simulink model "powerwindow_tl_v01"  (R2021a)
settings: Solver=ode1  StartTime=0.0  StopTime=20.0  FixedStep=0.01  RelTol=1e-3
PreLoadFcn:
  | if exist('tl_preloadfcn','file'), tl_preloadfcn(gcs,'22.1.0.27'); end
PostLoadFcn:
  | if exist('tl_postloadfcn','file'), tl_postloadfcn(gcs,'22.1.0.27'); end
InitFcn:
  | if exist('tlds_init','file'), tlds_init(gcs); end
StartFcn:
  | if exist('tlds_start','file'), tlds_start(gcs); end
StopFcn:
  | if exist('tlds_stop','file'), tlds_stop(gcs); end
undefined symbols (not defined in the file): auto_down_time, auto_up_time, emergency_down_time, position_endstop_top
libraries: tllib x7
(part 1 of 2)
PreSaveFcn:
  | if exist('tl_presavefcn','file'), tl_presavefcn(gcs); end
CloseFcn:
  | if exist('tl_closefcn','file'), tl_closefcn(gcs); end
settings Model: TL_MAIN_DATA={'codeopt',{'cleancode',1},'date',738946.6177900926,'advcodeopt',{'ExtendedBlockComments';'true'}}  DS_PROJECTFILE=powerwindow_tl_v01.dd  TLVersion=22.1.0.27  TL_GLOBAL_LOGGING_MODE=4  Creator=Wolfgang Meincke  LastModifiedBy=yatishc
settings SolverCC: AlgebraicLoopSolver=TrustRegion
settings DataIOCC: LimitDataPoints=on  SaveFormat=Array  ReturnWorkspaceOutputs=off
settings OptimizationCC: BlockReduction=off  BooleanDataType=off  ConditionallyExecuteInputs=off  OptimizeBlockIOStorage=off  BufferReuse=off  GlobalBufferReuse=off  ExpressionFolding=off  ExpressionDepthLimit=2147483647  LocalBlockOutputs=off  LifeSpan=inf  OptimizeDataStoreBuffers=off  BusAssignmentInplaceUpdate=off
settings DebuggingCC: SaveWithParameterizedLinksMsg=none  UnderspecifiedInitializationDetection=Classic  MergeDetectMultiDrivingBlocksExec=none  MultiTaskDSMMsg=warning  MultiTaskCondExecSysMsg=none  FcnCallInpInsideContextMsg=warning  UnconnectedInputMsg=none  UnconnectedOutputMsg=none  BusObjectLabelMismatch=error  StateNameClashWarn=warning  StrictBusMsg=ErrorOnBusTreatedAsVector  NonBusSignalsTreatedAsBus=error  SFUnexpectedBacktrackingDiag=warning  SFNoUnconditionalDefaultTransitionDiag=warning  SFMachineParentedDataDiag=warning  ArithmeticOperatorsInVariantConditions=warning
settings HardwareCC: ProdBitPerPointer=32  ProdBitPerSizeT=32  ProdBitPerPtrDiffT=32  ProdLargestAtomicFloat=None  ProdIntDivRoundTo=Undefined  ProdEndianess=Unspecified  ProdWordSize=32  ProdHWDeviceType=32-bit Generic
settings ModelReferenceCC: PropagateSignalLabelsOutOfModel=off
settings SFSimCC: SimUseLocalCustomCode=off  SimParseCustomCode=off  CustomCodeUndefinedFunction=UseInterfaceOnly
settings RTWCC: RTWUseLocalCustomCode=off
settings CodeAppCC: StateflowObjectComments=on
settings GRTTargetCC: TargetLangStandard=C89/C90 (ANSI)  CombineOutputUpdateFcns=off  GRTInterface=on
settings ConfigComp: CovMetricSettings=dw  CovSaveCumulativeToWorkspaceVar=on  CovSaveSingleToWorkspaceVar=on  CovExternalEMLEnable=off  CovSFcnEnable=off

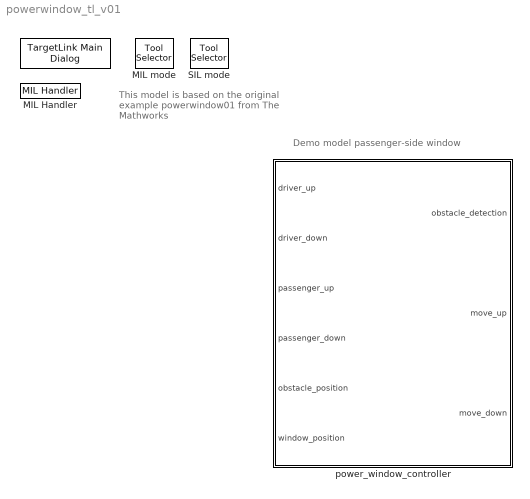
== system powerwindow_tl_v01 ==
  note: Demo model passenger-side window
  note: This model is based on the
      | original example powerwindow01
      | from The Mathworks
  " " : tllib/TargetLink Main Dialog  data=[]
      settings: SourceProductName=dSPACE TargetLink common blockset
  MIL Handler : tllib/MIL Handler  data={'date',730486}
      settings: SourceProductName=dSPACE TargetLink common blockset
  MIL mode : tllib/Tool Selector  Description=MIL\nmode  data={'date',730486}
      settings: SourceProductName=dSPACE TargetLink common blockset
  SIL mode : tllib/Tool Selector  Description=SIL\nmode  data={'date',730486}
      settings: SourceProductName=dSPACE TargetLink common blockset
  power_window_controller : Subsystem  Tag=TargetLink Simulation Frame  mask(TL_SimFrame){}
      settings: CopyFcn=if exist('tl_copyfcn','file'), tl_copyfcn(gcbh); end  NameChangeFcn=if exist('tl_framenamechangefcn','file'), tl_framenamechangefcn(gcbh); end
      settings: OpenFcn=|
      | if exist('open_tlsubsystem','file')
      |    open_tlsubsystem(gcbh);
      | else
      |    tlsubsystem = ...
      |       find_system(gcb, ...
      |       'LookUnderMasks','on', ...
      |       'FollowLinks','on', ...
      |       'Tag','MIL Subsystem');
      |    open_system(tlsubsystem);
      | end
      mask Display: disp('TargetLink\nModel-\nin-the-loop\nmode')

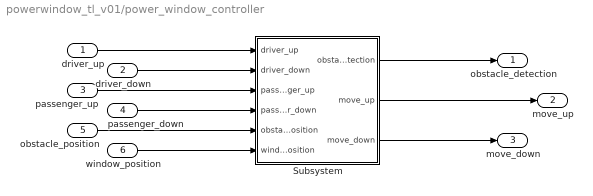
== system powerwindow_tl_v01/power_window_controller ==
  driver_up : Inport
  driver_down : Inport  Port=2
  passenger_up : Inport  Port=3
  passenger_down : Inport  Port=4
  obstacle_position : Inport  Port=5
  window_position : Inport  Port=6
  Subsystem : Subsystem  Tag=struct('sfcnName','power_window_controller_sf','subFunction','','srcSubsystem','')  mask(TL_Enable){}
      settings: OpenFcn=warndlg(get_param(gcb,'MaskHelp'),'Serious Warning');
      mask Help: This subsystem keeps the TargetLink subsystem (subsystem with TargetLink blocks for production code generation), and is needed for the TargetLink simulation frame to work properly. DO NOT DELETE OR MODIFY IT!
  obstacle_detection : Outport  VectorParamsAs1DForOutWhenUnconnected=off
  move_up : Outport  Port=2  VectorParamsAs1DForOutWhenUnconnected=off
  move_down : Outport  Port=3  VectorParamsAs1DForOutWhenUnconnected=off
  wires:
  driver_up/1 -> Subsystem/1(driver_up)
  driver_down/1 -> Subsystem/2(driver_down)
  passenger_up/1 -> Subsystem/3(passenger_up)
  passenger_down/1 -> Subsystem/4(passenger_down)
  obstacle_position/1 -> Subsystem/5(obstacle_position)
  window_position/1 -> Subsystem/6(window_position)
  Subsystem/1(obstacle_detection) -> obstacle_detection/1
  Subsystem/2(move_up) -> move_up/1
  Subsystem/3(move_down) -> move_down/1

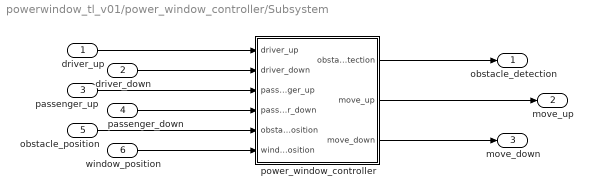
== system powerwindow_tl_v01/power_window_controller/Subsystem ==
  driver_up : Inport
  driver_down : Inport  Port=2
  passenger_up : Inport  Port=3
  passenger_down : Inport  Port=4
  obstacle_position : Inport  Port=5
  window_position : Inport  Port=6
  power_window_controller : Subsystem  Tag=MIL Subsystem  Description=a  RequirementInfo={} %GIDa_b80cfd7f_fc3d_42d1_9879_5951100bdf27  LoadFcn=|
      | if exist('TargetLink.SimFrameHandler.TLSubsystem','class')
      |     TargetLink.SimFrameHandler.TLSubsystem.CreateWatchDog(gcbh);
      | end
      settings: CopyFcn=if exist('tl_copyfcn','file'), tl_copyfcn(gcbh); end  NameChangeFcn=if exist('tl_namechangefcn','file'), tl_namechangefcn(gcbh); end  DestroyFcn=if exist('update_tl_main_dlg','file'), update_tl_main_dlg('TL_subs_display'); end
      mask Display: disp('TargetLink Subsystem')
  obstacle_detection : Outport  VectorParamsAs1DForOutWhenUnconnected=off
  move_up : Outport  Port=2  VectorParamsAs1DForOutWhenUnconnected=off
  move_down : Outport  Port=3  VectorParamsAs1DForOutWhenUnconnected=off
  wires:
  driver_up/1 -> power_window_controller/1(driver_up)
  driver_down/1 -> power_window_controller/2(driver_down)
  passenger_up/1 -> power_window_controller/3(passenger_up)
  passenger_down/1 -> power_window_controller/4(passenger_down)
  obstacle_position/1 -> power_window_controller/5(obstacle_position)
  window_position/1 -> power_window_controller/6(window_position)
  power_window_controller/1(obstacle_detection) -> obstacle_detection/1
  power_window_controller/2(move_up) -> move_up/1
  power_window_controller/3(move_down) -> move_down/1

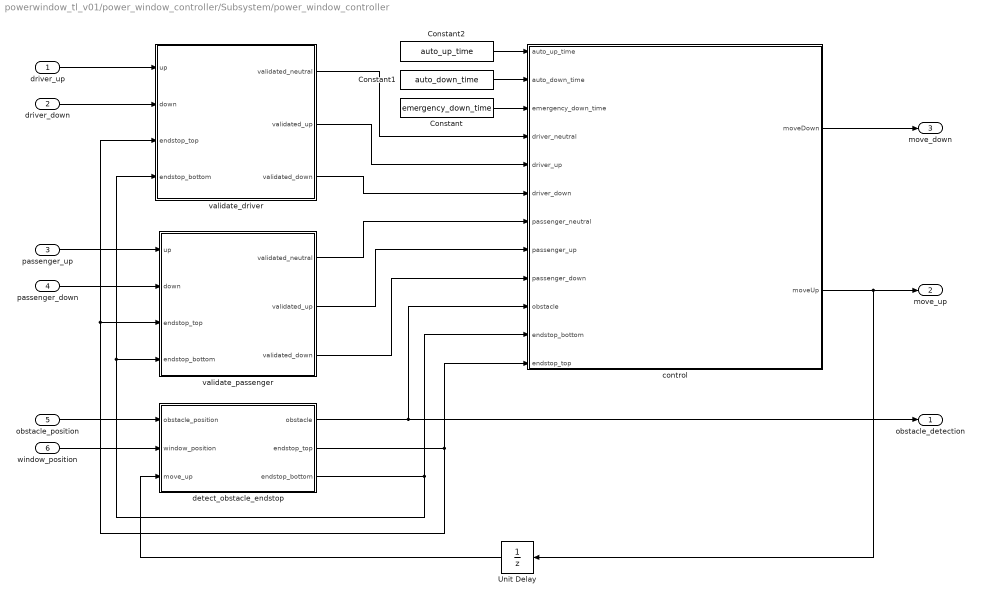
== system powerwindow_tl_v01/power_window_controller/Subsystem/power_window_controller ==
  driver_up : Inport  RequirementInfo={} %GIDa_750a3b1c_a79a_4067_88d9_431790a89f5d  PortDimensions=1  mask(TL_Inport){data={'output',{'variable','Interface_Variables/driver_up'},'date',737859.74382688652}}
      settings: CopyFcn=if exist('copy_tlblock','file')==2,copy_tlblock(gcbh);end  DeleteFcn=if exist('delete_tlblock','file')==2,delete_tlblock(gcbh);end  NameChangeFcn=if exist('rename_tlblock','file')==2,rename_tlblock(gcbh);end  OpenFcn=if exist('tl_open_blockdlg','file')==2,tl_open_blockdlg(gcbh);else,open_system(gcbh,'parameter');end
      mask Help: eval(['if exist(''tl_online_help'',''file'') == 2, tl_online_help(''Topic'',''TL_Inport''),else, web([''jar:file:///'',matlabroot,''/help/toolbox/simulink/help.jar!/slref/' lower(get_param(gcbh,'Blocktype')) '.html''], ''-helpbrowser''),end'])
      mask Display:
      | [x,y] = tlDrawBrandOnBlockIcon(gcbh);
      | plot(x,y);
  driver_down : Inport  RequirementInfo={} %GIDa_6d11f596_882a_4ff9_a83e_d4d289160ffc  Port=2  PortDimensions=1  mask(TL_Inport){data={'output',{'variable','Interface_Variables/driver_down'},'date',737859.74382813659}}
      settings: CopyFcn=if exist('copy_tlblock','file')==2,copy_tlblock(gcbh);end  DeleteFcn=if exist('delete_tlblock','file')==2,delete_tlblock(gcbh);end  NameChangeFcn=if exist('rename_tlblock','file')==2,rename_tlblock(gcbh);end  OpenFcn=if exist('tl_open_blockdlg','file')==2,tl_open_blockdlg(gcbh);else,open_system(gcbh,'parameter');end
      mask Help: eval(['if exist(''tl_online_help'',''file'') == 2, tl_online_help(''Topic'',''TL_Inport''),else, web([''jar:file:///'',matlabroot,''/help/toolbox/simulink/help.jar!/slref/' lower(get_param(gcbh,'Blocktype')) '.html''], ''-helpbrowser''),end'])
      mask Display:
      | [x,y] = tlDrawBrandOnBlockIcon(gcbh);
      | plot(x,y);
  passenger_up : Inport  RequirementInfo={} %GIDa_37c1ad15_e81b_4888_89b1_052434cfbb89  Port=3  PortDimensions=1  mask(TL_Inport){data={'output',{'variable','Interface_Variables/passenger_up'},'date',737859.74382853007}}
      settings: CopyFcn=if exist('copy_tlblock','file')==2,copy_tlblock(gcbh);end  DeleteFcn=if exist('delete_tlblock','file')==2,delete_tlblock(gcbh);end  NameChangeFcn=if exist('rename_tlblock','file')==2,rename_tlblock(gcbh);end  OpenFcn=if exist('tl_open_blockdlg','file')==2,tl_open_blockdlg(gcbh);else,open_system(gcbh,'parameter');end
      mask Help: eval(['if exist(''tl_online_help'',''file'') == 2, tl_online_help(''Topic'',''TL_Inport''),else, web([''jar:file:///'',matlabroot,''/help/toolbox/simulink/help.jar!/slref/' lower(get_param(gcbh,'Blocktype')) '.html''], ''-helpbrowser''),end'])
      mask Display:
      | [x,y] = tlDrawBrandOnBlockIcon(gcbh);
      | plot(x,y);
  passenger_down : Inport  RequirementInfo={} %GIDa_785e7f27_a7f1_4b54_8fd7_681828111c23  Port=4  PortDimensions=1  mask(TL_Inport){data={'output',{'variable','Interface_Variables/passenger_down'},'date',737859.74382914347}}
      settings: CopyFcn=if exist('copy_tlblock','file')==2,copy_tlblock(gcbh);end  DeleteFcn=if exist('delete_tlblock','file')==2,delete_tlblock(gcbh);end  NameChangeFcn=if exist('rename_tlblock','file')==2,rename_tlblock(gcbh);end  OpenFcn=if exist('tl_open_blockdlg','file')==2,tl_open_blockdlg(gcbh);else,open_system(gcbh,'parameter');end
      mask Help: eval(['if exist(''tl_online_help'',''file'') == 2, tl_online_help(''Topic'',''TL_Inport''),else, web([''jar:file:///'',matlabroot,''/help/toolbox/simulink/help.jar!/slref/' lower(get_param(gcbh,'Blocktype')) '.html''], ''-helpbrowser''),end'])
      mask Display:
      | [x,y] = tlDrawBrandOnBlockIcon(gcbh);
      | plot(x,y);
  obstacle_position : Inport  RequirementInfo={} %GIDa_c852d148_69a2_44b2_91eb_10d8d3731c30  Port=5  PortDimensions=1  mask(TL_Inport){data={'output',{'variable','Interface_Variables/obstacle_position'},'autoscaling',{'mode',0},'date',737869.45975795144}}
      settings: CopyFcn=if exist('copy_tlblock','file')==2,copy_tlblock(gcbh);end  DeleteFcn=if exist('delete_tlblock','file')==2,delete_tlblock(gcbh);end  NameChangeFcn=if exist('rename_tlblock','file')==2,rename_tlblock(gcbh);end  OpenFcn=if exist('tl_open_blockdlg','file')==2,tl_open_blockdlg(gcbh);else,open_system(gcbh,'parameter');end
      mask Help: eval(['if exist(''tl_online_help'',''file'') == 2, tl_online_help(''Topic'',''TL_Inport''),else, web([''jar:file:///'',matlabroot,''/help/toolbox/simulink/help.jar!/slref/' lower(get_param(gcbh,'Blocktype')) '.html''], ''-helpbrowser''),end'])
      mask Display:
      | [x,y] = tlDrawBrandOnBlockIcon(gcbh);
      | plot(x,y);
  window_position : Inport  RequirementInfo={} %GIDa_527401dc_d2fc_43f1_9503_1f5713b1657a  Port=6  PortDimensions=1  mask(TL_Inport){data={'output',{'variable','Interface_Variables/window_position'},'autoscaling',{'mode',0},'date',738946.61777480319}}
      settings: CopyFcn=if exist('copy_tlblock','file')==2,copy_tlblock(gcbh);end  DeleteFcn=if exist('delete_tlblock','file')==2,delete_tlblock(gcbh);end  NameChangeFcn=if exist('rename_tlblock','file')==2,rename_tlblock(gcbh);end  OpenFcn=if exist('tl_open_blockdlg','file')==2,tl_open_blockdlg(gcbh);else,open_system(gcbh,'parameter');end
      mask Help: eval(['if exist(''tl_online_help'',''file'') == 2, tl_online_help(''Topic'',''TL_Inport''),else, web([''jar:file:///'',matlabroot,''/help/toolbox/simulink/help.jar!/slref/' lower(get_param(gcbh,'Blocktype')) '.html''], ''-helpbrowser''),end'])
      mask Display:
      | [x,y] = tlDrawBrandOnBlockIcon(gcbh);
      | plot(x,y);
  Constant : Constant  RequirementInfo={} %GIDa_c9ec6c8d_2743_4165_a701_f3b966281310  Value=emergency_down_time  mask(TL_Constant){data={'output',{'variable','Parameter/emergency_down_time'},'date',735993.41955673613}}
      settings: CopyFcn=if exist('copy_tlblock','file')==2,copy_tlblock(gcbh);end  DeleteFcn=if exist('delete_tlblock','file')==2,delete_tlblock(gcbh);end  NameChangeFcn=if exist('rename_tlblock','file')==2,rename_tlblock(gcbh);end  OpenFcn=if exist('tl_open_blockdlg','file')==2,tl_open_blockdlg(gcbh);else,open_system(gcbh,'parameter');end
      mask Help: eval(['if exist(''tl_online_help'',''file'') == 2, tl_online_help(''Topic'',''TL_Constant''),else, web([''jar:file:///'',matlabroot,''/help/toolbox/simulink/help.jar!/slref/' lower(get_param(gcbh,'Blocktype')) '.html''], ''-helpbrowser''),end'])
      mask Display:
      | [x,y] = tlDrawBrandOnBlockIcon(gcbh);
      | plot(x,y);
  Constant1 : Constant  RequirementInfo={} %GIDa_5bcfbdf2_6dc9_458c_8155_820a7ffe3dc3  Value=auto_down_time  mask(TL_Constant){data={'output',{'variable','Parameter/auto_down_time'},'date',735993.41940997681}}
      settings: CopyFcn=if exist('copy_tlblock','file')==2,copy_tlblock(gcbh);end  DeleteFcn=if exist('delete_tlblock','file')==2,delete_tlblock(gcbh);end  NameChangeFcn=if exist('rename_tlblock','file')==2,rename_tlblock(gcbh);end  OpenFcn=if exist('tl_open_blockdlg','file')==2,tl_open_blockdlg(gcbh);else,open_system(gcbh,'parameter');end
      mask Help: eval(['if exist(''tl_online_help'',''file'') == 2, tl_online_help(''Topic'',''TL_Constant''),else, web([''jar:file:///'',matlabroot,''/help/toolbox/simulink/help.jar!/slref/' lower(get_param(gcbh,'Blocktype')) '.html''], ''-helpbrowser''),end'])
      mask Display:
      | [x,y] = tlDrawBrandOnBlockIcon(gcbh);
      | plot(x,y);
  Constant2 : Constant  RequirementInfo={} %GIDa_904ec5cd_79a7_49d7_a756_f8f2caa0ffb6  Value=auto_up_time  mask(TL_Constant){data={'output',{'variable','Parameter/auto_up_time'},'date',735993.41923796292}}
      settings: CopyFcn=if exist('copy_tlblock','file')==2,copy_tlblock(gcbh);end  DeleteFcn=if exist('delete_tlblock','file')==2,delete_tlblock(gcbh);end  NameChangeFcn=if exist('rename_tlblock','file')==2,rename_tlblock(gcbh);end  OpenFcn=if exist('tl_open_blockdlg','file')==2,tl_open_blockdlg(gcbh);else,open_system(gcbh,'parameter');end
      mask Help: eval(['if exist(''tl_online_help'',''file'') == 2, tl_online_help(''Topic'',''TL_Constant''),else, web([''jar:file:///'',matlabroot,''/help/toolbox/simulink/help.jar!/slref/' lower(get_param(gcbh,'Blocktype')) '.html''], ''-helpbrowser''),end'])
      mask Display:
      | [x,y] = tlDrawBrandOnBlockIcon(gcbh);
      | plot(x,y);
  Unit Delay : UnitDelay  RequirementInfo={} %GIDa_482e15a8_f012_4ab2_9ff3_fdc6f4763625  SampleTime=-1  HasFrameUpgradeWarning=on  mask(TL_UnitDelay){data={'output',{'inheritscaling',1},'date',735992.65481520828}}
      settings: CopyFcn=if exist('copy_tlblock','file')==2,copy_tlblock(gcbh);end  DeleteFcn=if exist('delete_tlblock','file')==2,delete_tlblock(gcbh);end  NameChangeFcn=if exist('rename_tlblock','file')==2,rename_tlblock(gcbh);end  OpenFcn=if exist('tl_open_blockdlg','file')==2,tl_open_blockdlg(gcbh);else,open_system(gcbh,'parameter');end
      mask Help: eval(['if exist(''tl_online_help'',''file'') == 2, tl_online_help(''Topic'',''TL_UnitDelay''),else, web([''jar:file:///'',matlabroot,''/help/toolbox/simulink/help.jar!/slref/' lower(get_param(gcbh,'Blocktype')) '.html''], ''-helpbrowser''),end'])
      mask Display:
      | [x,y] = tlDrawBrandOnBlockIcon(gcbh);
      | plot(x,y);
  control : Stateflow chart  RequirementInfo={} %GIDa_7d3839c0_ef15_4391_a968_14c5965a3773  TreatAsAtomicUnit=on
  detect_obstacle_endstop : Subsystem  RequirementInfo={} %GIDa_8885f1ca_0ce8_4b9c_95ac_ca70d8939616  TreatAsAtomicUnit=on
  validate_driver : Subsystem  RequirementInfo={} %GIDa_1aa80d5b_b151_4f2e_b721_8678ee4b3aef  TreatAsAtomicUnit=on
  validate_passenger : Subsystem  RequirementInfo={} %GIDa_2761634b_047a_4d48_9f8a_6da147749019  TreatAsAtomicUnit=on
  obstacle_detection : Outport  RequirementInfo={} %GIDa_144c3af4_9b2f_4012_866c_c128ef723a51  PortDimensions=1  VectorParamsAs1DForOutWhenUnconnected=off  mask(TL_Outport){data={'output',{'variable','Interface_Variables/obstacle_detection'},'date',737859.74383184023}}
      settings: CopyFcn=if exist('copy_tlblock','file')==2,copy_tlblock(gcbh);end  DeleteFcn=if exist('delete_tlblock','file')==2,delete_tlblock(gcbh);end  NameChangeFcn=if exist('rename_tlblock','file')==2,rename_tlblock(gcbh);end  OpenFcn=if exist('tl_open_blockdlg','file')==2,tl_open_blockdlg(gcbh);else,open_system(gcbh,'parameter');end
      mask Help: eval(['if exist(''tl_online_help'',''file'') == 2, tl_online_help(''Topic'',''TL_Outport''),else, web([''jar:file:///'',matlabroot,''/help/toolbox/simulink/help.jar!/slref/' lower(get_param(gcbh,'Blocktype')) '.html''], ''-helpbrowser''),end'])
      mask Display:
      | [x,y] = tlDrawBrandOnBlockIcon(gcbh);
      | plot(x,y);
  move_up : Outport  RequirementInfo={} %GIDa_74f6944e_1281_467d_a8a8_9ff5463f9340  Port=2  PortDimensions=1  VectorParamsAs1DForOutWhenUnconnected=off  mask(TL_Outport){data={'output',{'variable','Interface_Variables/move_up'},'date',738946.61777651624}}
      settings: CopyFcn=if exist('copy_tlblock','file')==2,copy_tlblock(gcbh);end  DeleteFcn=if exist('delete_tlblock','file')==2,delete_tlblock(gcbh);end  NameChangeFcn=if exist('rename_tlblock','file')==2,rename_tlblock(gcbh);end  OpenFcn=if exist('tl_open_blockdlg','file')==2,tl_open_blockdlg(gcbh);else,open_system(gcbh,'parameter');end
      mask Help: eval(['if exist(''tl_online_help'',''file'') == 2, tl_online_help(''Topic'',''TL_Outport''),else, web([''jar:file:///'',matlabroot,''/help/toolbox/simulink/help.jar!/slref/' lower(get_param(gcbh,'Blocktype')) '.html''], ''-helpbrowser''),end'])
      mask Display:
      | [x,y] = tlDrawBrandOnBlockIcon(gcbh);
      | plot(x,y);
  move_down : Outport  RequirementInfo={} %GIDa_b32d78ce_e749_48bf_8460_9dfb4f3d1222  Port=3  PortDimensions=1  VectorParamsAs1DForOutWhenUnconnected=off  mask(TL_Outport){data={'output',{'variable','Interface_Variables/move_down'},'date',738946.61777693289}}
      settings: CopyFcn=if exist('copy_tlblock','file')==2,copy_tlblock(gcbh);end  DeleteFcn=if exist('delete_tlblock','file')==2,delete_tlblock(gcbh);end  NameChangeFcn=if exist('rename_tlblock','file')==2,rename_tlblock(gcbh);end  OpenFcn=if exist('tl_open_blockdlg','file')==2,tl_open_blockdlg(gcbh);else,open_system(gcbh,'parameter');end
      mask Help: eval(['if exist(''tl_online_help'',''file'') == 2, tl_online_help(''Topic'',''TL_Outport''),else, web([''jar:file:///'',matlabroot,''/help/toolbox/simulink/help.jar!/slref/' lower(get_param(gcbh,'Blocktype')) '.html''], ''-helpbrowser''),end'])
      mask Display:
      | [x,y] = tlDrawBrandOnBlockIcon(gcbh);
      | plot(x,y);
  wires:
  detect_obstacle_endstop/3(endstop_bottom) -> validate_passenger/4(endstop_bottom), validate_driver/4(endstop_bottom), control/11(endstop_bottom)
  detect_obstacle_endstop/2(endstop_top) -> validate_passenger/3(endstop_top), validate_driver/3(endstop_top), control/12(endstop_top)
  validate_passenger/3(validated_down) -> control/9(passenger_down)
  validate_passenger/2(validated_up) -> control/8(passenger_up)
  validate_passenger/1(validated_neutral) -> control/7(passenger_neutral)
  validate_driver/3(validated_down) -> control/6(driver_down)
  validate_driver/2(validated_up) -> control/5(driver_up)
  validate_driver/1(validated_neutral) -> control/4(driver_neutral)
  Constant/1 -> control/3(emergency_down_time)
  Constant1/1 -> control/2(auto_down_time)
  Constant2/1 -> control/1(auto_up_time)
  control/1(moveDown) -> move_down/1
  control/2(moveUp) -> Unit Delay/1, move_up/1
  detect_obstacle_endstop/1(obstacle) -> control/10(obstacle), obstacle_detection/1
  Unit Delay/1 -> detect_obstacle_endstop/3(move_up)
  window_position/1 -> detect_obstacle_endstop/2(window_position)
  obstacle_position/1 -> detect_obstacle_endstop/1(obstacle_position)
  passenger_down/1 -> validate_passenger/2(down)
  passenger_up/1 -> validate_passenger/1(up)
  driver_down/1 -> validate_driver/2(down)
  driver_up/1 -> validate_driver/1(up)

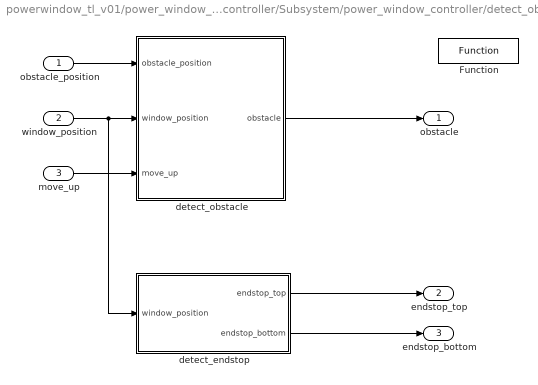
== system powerwindow_tl_v01/power_window_controller/Subsystem/power_window_controller/detect_obstacle_endstop ==
  obstacle_position : Inport  RequirementInfo={} %GIDa_6425afca_4bc7_4317_9760_19aaa65339cd  mask(TL_Inport){data={'output',{'class','FCN_ARG','type','UInt16','scaling','position'},'autoscaling',{'mode',0},'date',737859.74382997688}}
      settings: CopyFcn=if exist('copy_tlblock','file')==2,copy_tlblock(gcbh);end  DeleteFcn=if exist('delete_tlblock','file')==2,delete_tlblock(gcbh);end  NameChangeFcn=if exist('rename_tlblock','file')==2,rename_tlblock(gcbh);end  OpenFcn=if exist('tl_open_blockdlg','file')==2,tl_open_blockdlg(gcbh);else,open_system(gcbh,'parameter');end
      mask Help: eval(['if exist(''tl_online_help'',''file'') == 2, tl_online_help(''Topic'',''TL_Inport''),else, web([''jar:file:///'',matlabroot,''/help/toolbox/simulink/help.jar!/slref/' lower(get_param(gcbh,'Blocktype')) '.html''], ''-helpbrowser''),end'])
      mask Display:
      | [x,y] = tlDrawBrandOnBlockIcon(gcbh);
      | plot(x,y);
  window_position : Inport  RequirementInfo={} %GIDa_a332e1d1_0df8_4eb0_a712_106cdf854f9a  Port=2  mask(TL_Inport){data={'output',{'max',0.45,'min',0,'class','FCN_ARG','type','UInt8','scaling','position'},'autoscaling',{'mode',0},'date',737859.74766700226}}
      settings: CopyFcn=if exist('copy_tlblock','file')==2,copy_tlblock(gcbh);end  DeleteFcn=if exist('delete_tlblock','file')==2,delete_tlblock(gcbh);end  NameChangeFcn=if exist('rename_tlblock','file')==2,rename_tlblock(gcbh);end  OpenFcn=if exist('tl_open_blockdlg','file')==2,tl_open_blockdlg(gcbh);else,open_system(gcbh,'parameter');end
      mask Help: eval(['if exist(''tl_online_help'',''file'') == 2, tl_online_help(''Topic'',''TL_Inport''),else, web([''jar:file:///'',matlabroot,''/help/toolbox/simulink/help.jar!/slref/' lower(get_param(gcbh,'Blocktype')) '.html''], ''-helpbrowser''),end'])
      mask Display:
      | [x,y] = tlDrawBrandOnBlockIcon(gcbh);
      | plot(x,y);
  move_up : Inport  RequirementInfo={} %GIDa_de64c120_4c5c_45bf_9859_8bab9597cbad  Port=3  mask(TL_Inport){data={'output',{'class','FCN_ARG','type','Bool'},'date',737859.74383032403}}
      settings: CopyFcn=if exist('copy_tlblock','file')==2,copy_tlblock(gcbh);end  DeleteFcn=if exist('delete_tlblock','file')==2,delete_tlblock(gcbh);end  NameChangeFcn=if exist('rename_tlblock','file')==2,rename_tlblock(gcbh);end  OpenFcn=if exist('tl_open_blockdlg','file')==2,tl_open_blockdlg(gcbh);else,open_system(gcbh,'parameter');end
      mask Help: eval(['if exist(''tl_online_help'',''file'') == 2, tl_online_help(''Topic'',''TL_Inport''),else, web([''jar:file:///'',matlabroot,''/help/toolbox/simulink/help.jar!/slref/' lower(get_param(gcbh,'Blocktype')) '.html''], ''-helpbrowser''),end'])
      mask Display:
      | [x,y] = tlDrawBrandOnBlockIcon(gcbh);
      | plot(x,y);
  Function : tllib/Function  RequirementInfo={} %GIDa_a41663b0_75ca_4be6_8eec_cc6cae1c742b  data={'stepfunctionname','$B','codefile','$B','date',737859.74383232638}  displayString=FUNCTION
      settings: SourceProductName=dSPACE TargetLink common blockset
  detect_endstop : Subsystem  RequirementInfo={} %GIDa_c4862fce_da6b_429c_87a7_fab53ca25f21
  detect_obstacle : Subsystem  RequirementInfo={} %GIDa_821ba426_233a_44e7_910d_06f90508fb41
  obstacle : Outport  RequirementInfo={} %GIDa_25467cbe_d28b_429d_8008_370fc26ef791  VectorParamsAs1DForOutWhenUnconnected=off  mask(TL_Outport){data={'output',{'type','Bool'},'date',737859.74383100693}}
      settings: CopyFcn=if exist('copy_tlblock','file')==2,copy_tlblock(gcbh);end  DeleteFcn=if exist('delete_tlblock','file')==2,delete_tlblock(gcbh);end  NameChangeFcn=if exist('rename_tlblock','file')==2,rename_tlblock(gcbh);end  OpenFcn=if exist('tl_open_blockdlg','file')==2,tl_open_blockdlg(gcbh);else,open_system(gcbh,'parameter');end
      mask Help: eval(['if exist(''tl_online_help'',''file'') == 2, tl_online_help(''Topic'',''TL_Outport''),else, web([''jar:file:///'',matlabroot,''/help/toolbox/simulink/help.jar!/slref/' lower(get_param(gcbh,'Blocktype')) '.html''], ''-helpbrowser''),end'])
      mask Display:
      | [x,y] = tlDrawBrandOnBlockIcon(gcbh);
      | plot(x,y);
  endstop_top : Outport  RequirementInfo={} %GIDa_0bf4bf11_d8c1_4837_94da_fc152485df5a  Port=2  VectorParamsAs1DForOutWhenUnconnected=off  mask(TL_Outport){data={'output',{'type','Bool'},'date',737859.74383120367}}
      settings: CopyFcn=if exist('copy_tlblock','file')==2,copy_tlblock(gcbh);end  DeleteFcn=if exist('delete_tlblock','file')==2,delete_tlblock(gcbh);end  NameChangeFcn=if exist('rename_tlblock','file')==2,rename_tlblock(gcbh);end  OpenFcn=if exist('tl_open_blockdlg','file')==2,tl_open_blockdlg(gcbh);else,open_system(gcbh,'parameter');end
      mask Help: eval(['if exist(''tl_online_help'',''file'') == 2, tl_online_help(''Topic'',''TL_Outport''),else, web([''jar:file:///'',matlabroot,''/help/toolbox/simulink/help.jar!/slref/' lower(get_param(gcbh,'Blocktype')) '.html''], ''-helpbrowser''),end'])
      mask Display:
      | [x,y] = tlDrawBrandOnBlockIcon(gcbh);
      | plot(x,y);
  endstop_bottom : Outport  RequirementInfo={} %GIDa_2dd66280_08c4_4121_9342_4562e20f164c  Port=3  VectorParamsAs1DForOutWhenUnconnected=off  mask(TL_Outport){data={'output',{'type','Bool'},'date',737859.74383136572}}
      settings: CopyFcn=if exist('copy_tlblock','file')==2,copy_tlblock(gcbh);end  DeleteFcn=if exist('delete_tlblock','file')==2,delete_tlblock(gcbh);end  NameChangeFcn=if exist('rename_tlblock','file')==2,rename_tlblock(gcbh);end  OpenFcn=if exist('tl_open_blockdlg','file')==2,tl_open_blockdlg(gcbh);else,open_system(gcbh,'parameter');end
      mask Help: eval(['if exist(''tl_online_help'',''file'') == 2, tl_online_help(''Topic'',''TL_Outport''),else, web([''jar:file:///'',matlabroot,''/help/toolbox/simulink/help.jar!/slref/' lower(get_param(gcbh,'Blocktype')) '.html''], ''-helpbrowser''),end'])
      mask Display:
      | [x,y] = tlDrawBrandOnBlockIcon(gcbh);
      | plot(x,y);
  wires:
  detect_endstop/2(endstop_bottom) -> endstop_bottom/1
  detect_endstop/1(endstop_top) -> endstop_top/1
  detect_obstacle/1(obstacle) -> obstacle/1
  obstacle_position/1 -> detect_obstacle/1(obstacle_position)
  window_position/1 -> detect_endstop/1(window_position), detect_obstacle/2(window_position)
  move_up/1 -> detect_obstacle/3(move_up)

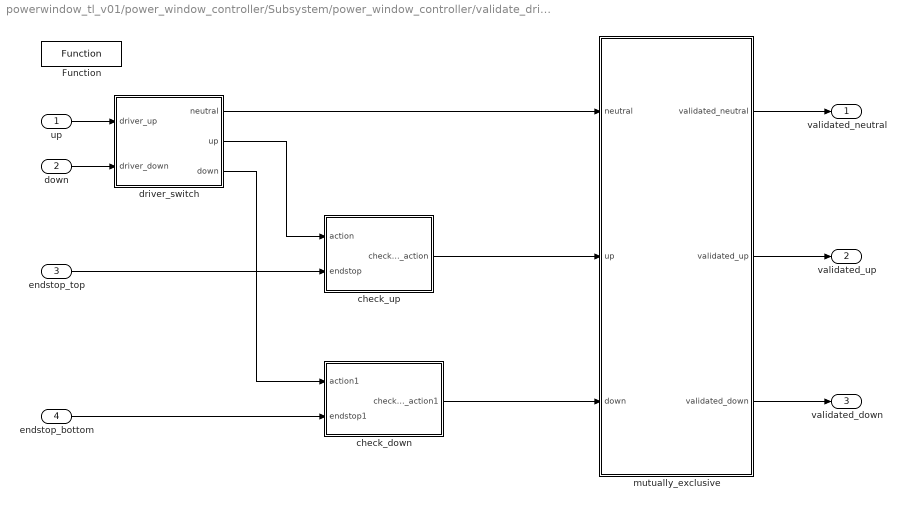
== system powerwindow_tl_v01/power_window_controller/Subsystem/power_window_controller/validate_driver ==
  up : Inport  RequirementInfo={} %GIDa_3ec099f3_6205_46c9_a44d_f051e8db2f47
  down : Inport  RequirementInfo={} %GIDa_f444f593_8241_4dc8_9a71_91d7b4c463c7  Port=2
  endstop_top : Inport  RequirementInfo={} %GIDa_e1a93f72_f94c_46cc_a369_7235f4f9911c  Port=3
  endstop_bottom : Inport  RequirementInfo={} %GIDa_4177fe9e_66e3_4618_a797_fa77e200eb5f  Port=4
  Function : tllib/Function  RequirementInfo={} %GIDa_4283c40f_4de8_4c99_ae32_2ee78f222cb2  data={'stepfunctionname','$B','codefile','$B','date',737859.74383252312}  displayString=FUNCTION
      settings: SourceProductName=dSPACE TargetLink common blockset
  check_down : Subsystem  RequirementInfo={} %GIDa_2a134998_5b68_4c38_994a_71b9de565b5a
  check_up : Subsystem  RequirementInfo={} %GIDa_252fa563_8156_43ee_ae73_fa7ef79d35b6
  driver_switch : Subsystem  RequirementInfo={} %GIDa_680e2dda_7223_4722_a747_c5766ffd315d
  mutually_exclusive : Subsystem  RequirementInfo={} %GIDa_e4ed0248_1aae_477c_a870_d3fc645b3c6f
  validated_neutral : Outport  RequirementInfo={} %GIDa_4af49be8_1940_40e2_a47c_487cbecf9e02  VectorParamsAs1DForOutWhenUnconnected=off
  validated_up : Outport  RequirementInfo={} %GIDa_0e41dc29_c372_48d7_a532_9bf74d08c1e5  Port=2  VectorParamsAs1DForOutWhenUnconnected=off
  validated_down : Outport  RequirementInfo={} %GIDa_fad4bf66_52bd_4a4e_9fec_f9cf878f0919  Port=3  VectorParamsAs1DForOutWhenUnconnected=off
  wires:
  mutually_exclusive/3(validated_down) -> validated_down/1
  mutually_exclusive/2(validated_up) -> validated_up/1
  mutually_exclusive/1(validated_neutral) -> validated_neutral/1
  check_down/1(checked_action1) -> mutually_exclusive/3(down)
  check_up/1(checked_action) -> mutually_exclusive/2(up)
  driver_switch/1(neutral) -> mutually_exclusive/1(neutral)
  endstop_bottom/1 -> check_down/2(endstop1)
  endstop_top/1 -> check_up/2(endstop)
  driver_switch/3(down) -> check_down/1(action1)
  driver_switch/2(up) -> check_up/1(action)
  down/1 -> driver_switch/2(driver_down)
  up/1 -> driver_switch/1(driver_up)

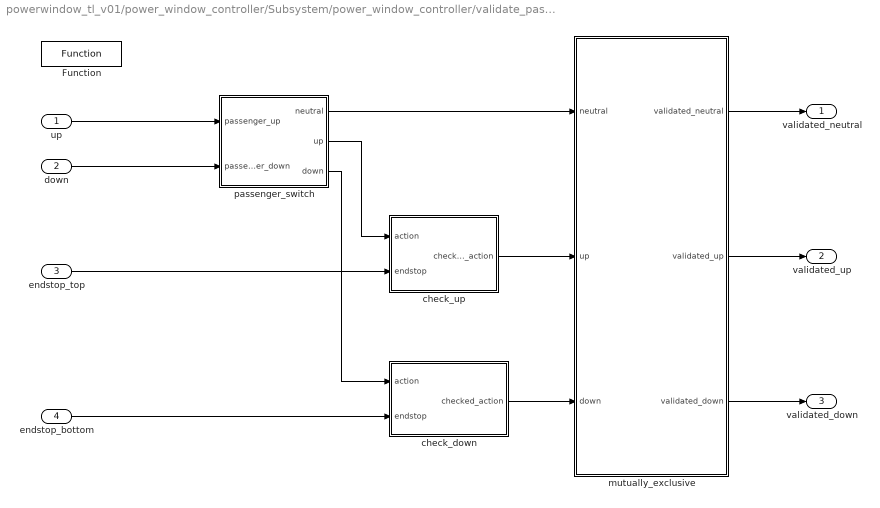
== system powerwindow_tl_v01/power_window_controller/Subsystem/power_window_controller/validate_passenger ==
  up : Inport  RequirementInfo={} %GIDa_6f1af6f1_1d88_4512_bf37_00203feafbc6
  down : Inport  RequirementInfo={} %GIDa_dc205db0_683d_43a8_9125_281867d44e02  Port=2
  endstop_top : Inport  RequirementInfo={} %GIDa_68e970db_4102_44cd_85e0_584f2744f5b5  Port=3
  endstop_bottom : Inport  RequirementInfo={} %GIDa_e1b42b93_0686_4386_a420_6729e763e78e  Port=4
  Function : tllib/Function  RequirementInfo={} %GIDa_d9bdec14_8517_40fa_b916_161616e78022  data={'stepfunctionname','$B','codefile','$B','date',737859.74383277772}  displayString=FUNCTION
      settings: SourceProductName=dSPACE TargetLink common blockset
  check_down : Subsystem  RequirementInfo={} %GIDa_13ac8a74_9456_4adf_ae7c_643bb7998cf8
  check_up : Subsystem  RequirementInfo={} %GIDa_bf523630_09b4_4ad3_bd02_e66063895e8a
  mutually_exclusive : Subsystem  RequirementInfo={} %GIDa_9a239d5b_a3b0_4ee9_bec6_4441f8275b5f
  passenger_switch : Subsystem  RequirementInfo={} %GIDa_387b2ef4_d57f_4698_b5b1_c6cb3d950432
  validated_neutral : Outport  RequirementInfo={} %GIDa_7acf03f3_93cb_4f80_bf7c_c44cdc63f879  VectorParamsAs1DForOutWhenUnconnected=off
  validated_up : Outport  RequirementInfo={} %GIDa_2aee5fa1_4546_4cd7_8a39_591316a723f8  Port=2  VectorParamsAs1DForOutWhenUnconnected=off
  validated_down : Outport  RequirementInfo={} %GIDa_c6e8d142_9084_420b_8967_e24ac98e1973  Port=3  VectorParamsAs1DForOutWhenUnconnected=off
  wires:
  mutually_exclusive/3(validated_down) -> validated_down/1
  mutually_exclusive/2(validated_up) -> validated_up/1
  mutually_exclusive/1(validated_neutral) -> validated_neutral/1
  check_down/1(checked_action) -> mutually_exclusive/3(down)
  check_up/1(checked_action) -> mutually_exclusive/2(up)
  passenger_switch/1(neutral) -> mutually_exclusive/1(neutral)
  endstop_bottom/1 -> check_down/2(endstop)
  endstop_top/1 -> check_up/2(endstop)
  passenger_switch/3(down) -> check_down/1(action)
  passenger_switch/2(up) -> check_up/1(action)
  down/1 -> passenger_switch/2(passenger_down)
  up/1 -> passenger_switch/1(passenger_up)

== system powerwindow_tl_v01/power_window_controller/Subsystem/power_window_controller/detect_obstacle_endstop/detect_endstop ==
  window_position : Inport  RequirementInfo={} %GIDa_9ee00257_4db9_4855_9723_23935ff30e16
  "Constant " : Constant  RequirementInfo={} %GIDa_8ba3300b_17d3_45c6_8e79_208caca35c19  Value=position_endstop_top  mask(TL_Constant){data={'output',{'variable','Parameter/position_endstop_top'},'date',735993.42899643513}}
      settings: CopyFcn=if exist('copy_tlblock','file')==2,copy_tlblock(gcbh);end  DeleteFcn=if exist('delete_tlblock','file')==2,delete_tlblock(gcbh);end  NameChangeFcn=if exist('rename_tlblock','file')==2,rename_tlblock(gcbh);end  OpenFcn=if exist('tl_open_blockdlg','file')==2,tl_open_blockdlg(gcbh);else,open_system(gcbh,'parameter');end
      mask Help: eval(['if exist(''tl_online_help'',''file'') == 2, tl_online_help(''Topic'',''TL_Constant''),else, web([''jar:file:///'',matlabroot,''/help/toolbox/simulink/help.jar!/slref/' lower(get_param(gcbh,'Blocktype')) '.html''], ''-helpbrowser''),end'])
      mask Display:
      | [x,y] = tlDrawBrandOnBlockIcon(gcbh);
      | plot(x,y);
  detection_endstop_bottom : RelationalOperator  RequirementInfo={} %GIDa_3ca3bec3_b611_44fd_88a7_7f551d16d954  Operator=<=  OutDataTypeStr=boolean  RndMeth=Nearest  mask(TL_RelationalOperator){data={'output',{'variable','Internal_Variables/detection_endstop_bottom'},'date',738946.61777771986}}
      settings: CopyFcn=if exist('copy_tlblock','file')==2,copy_tlblock(gcbh);end  DeleteFcn=if exist('delete_tlblock','file')==2,delete_tlblock(gcbh);end  NameChangeFcn=if exist('rename_tlblock','file')==2,rename_tlblock(gcbh);end  OpenFcn=if exist('tl_open_blockdlg','file')==2,tl_open_blockdlg(gcbh);else,open_system(gcbh,'parameter');end
      mask Help: eval(['if exist(''tl_online_help'',''file'') == 2, tl_online_help(''Topic'',''TL_RelationalOperator''),else, web([''jar:file:///'',matlabroot,''/help/toolbox/simulink/help.jar!/slref/' lower(get_param(gcbh,'Blocktype')) '.html''], ''-helpbrowser''),end'])
      mask Display:
      | [x,y] = tlDrawBrandOnBlockIcon(gcbh);
      | plot(x,y);
  detection_endstop_top : RelationalOperator  RequirementInfo={} %GIDa_e47f5b02_5693_4606_85da_ade41505839a  OutDataTypeStr=boolean  RndMeth=Nearest  mask(TL_RelationalOperator){data={'output',{'variable','Internal_Variables/detection_endstop_top'},'date',738946.61777799763}}
      settings: CopyFcn=if exist('copy_tlblock','file')==2,copy_tlblock(gcbh);end  DeleteFcn=if exist('delete_tlblock','file')==2,delete_tlblock(gcbh);end  NameChangeFcn=if exist('rename_tlblock','file')==2,rename_tlblock(gcbh);end  OpenFcn=if exist('tl_open_blockdlg','file')==2,tl_open_blockdlg(gcbh);else,open_system(gcbh,'parameter');end
      mask Help: eval(['if exist(''tl_online_help'',''file'') == 2, tl_online_help(''Topic'',''TL_RelationalOperator''),else, web([''jar:file:///'',matlabroot,''/help/toolbox/simulink/help.jar!/slref/' lower(get_param(gcbh,'Blocktype')) '.html''], ''-helpbrowser''),end'])
      mask Display:
      | [x,y] = tlDrawBrandOnBlockIcon(gcbh);
      | plot(x,y);
  position_endstop_bottom : Constant  RequirementInfo={} %GIDa_ad5aa93c_0ba5_4f5c_b2b9_2b42c9b6ab6c  Value=0  mask(TL_Constant){data={'date',735992.66554090276}}
      settings: CopyFcn=if exist('copy_tlblock','file')==2,copy_tlblock(gcbh);end  DeleteFcn=if exist('delete_tlblock','file')==2,delete_tlblock(gcbh);end  NameChangeFcn=if exist('rename_tlblock','file')==2,rename_tlblock(gcbh);end  OpenFcn=if exist('tl_open_blockdlg','file')==2,tl_open_blockdlg(gcbh);else,open_system(gcbh,'parameter');end
      mask Help: eval(['if exist(''tl_online_help'',''file'') == 2, tl_online_help(''Topic'',''TL_Constant''),else, web([''jar:file:///'',matlabroot,''/help/toolbox/simulink/help.jar!/slref/' lower(get_param(gcbh,'Blocktype')) '.html''], ''-helpbrowser''),end'])
      mask Display:
      | [x,y] = tlDrawBrandOnBlockIcon(gcbh);
      | plot(x,y);
  endstop_top : Outport  RequirementInfo={} %GIDa_149fe6d9_58f7_4e99_b04a_ce3ee20bf1c8  VectorParamsAs1DForOutWhenUnconnected=off
  endstop_bottom : Outport  RequirementInfo={} %GIDa_e6d43da9_9a07_4843_b09a_3f721bb4355d  Port=2  VectorParamsAs1DForOutWhenUnconnected=off
  wires:
  detection_endstop_bottom/1 -> endstop_bottom/1  "endstop_bottom"
  detection_endstop_top/1 -> endstop_top/1  "endstop_top"
  position_endstop_bottom/1 -> detection_endstop_bottom/2
  window_position/1 -> detection_endstop_bottom/1, detection_endstop_top/1
  "Constant "/1 -> detection_endstop_top/2

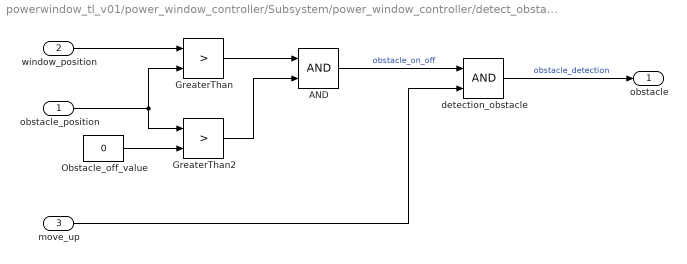
== system powerwindow_tl_v01/power_window_controller/Subsystem/power_window_controller/detect_obstacle_endstop/detect_obstacle ==
  obstacle_position : Inport  RequirementInfo={} %GIDa_802734e1_2062_4a38_ab79_1d79efc8a064
  window_position : Inport  RequirementInfo={} %GIDa_538c1468_0908_44cc_86e1_c376fd70aa70  Port=2
  move_up : Inport  RequirementInfo={} %GIDa_d28ded91_598e_4acd_a941_6f94a9e18b21  Port=3
  AND : Logic  RequirementInfo={} %GIDa_eb226a0d_2994_4da5_ac66_d2a839ff2ec3  AllPortsSameDT=off  OutDataTypeStr=boolean  mask(TL_LogicalOperator){data={'date',730486}}
      settings: CopyFcn=if exist('copy_tlblock','file')==2,copy_tlblock(gcbh);end  DeleteFcn=if exist('delete_tlblock','file')==2,delete_tlblock(gcbh);end  NameChangeFcn=if exist('rename_tlblock','file')==2,rename_tlblock(gcbh);end  OpenFcn=if exist('tl_open_blockdlg','file')==2,tl_open_blockdlg(gcbh);else,open_system(gcbh,'parameter');end
      mask Help: eval(['if exist(''tl_online_help'',''file'') == 2, tl_online_help(''Topic'',''TL_LogicalOperator''),else, web([''jar:file:///'',matlabroot,''/help/toolbox/simulink/help.jar!/slref/' lower(get_param(gcbh,'Blocktype')) '.html''], ''-helpbrowser''),end'])
      mask Display:
      | [x,y] = tlDrawBrandOnBlockIcon(gcbh);
      | plot(x,y);
  GreaterThan : RelationalOperator  RequirementInfo={} %GIDa_61fb225a_ac37_40fe_8ee6_258c4a11fd5b  Operator=>  OutDataTypeStr=boolean  RndMeth=Nearest  mask(TL_RelationalOperator){data={'date',735992.6592954282}}
      settings: CopyFcn=if exist('copy_tlblock','file')==2,copy_tlblock(gcbh);end  DeleteFcn=if exist('delete_tlblock','file')==2,delete_tlblock(gcbh);end  NameChangeFcn=if exist('rename_tlblock','file')==2,rename_tlblock(gcbh);end  OpenFcn=if exist('tl_open_blockdlg','file')==2,tl_open_blockdlg(gcbh);else,open_system(gcbh,'parameter');end
      mask Help: eval(['if exist(''tl_online_help'',''file'') == 2, tl_online_help(''Topic'',''TL_RelationalOperator''),else, web([''jar:file:///'',matlabroot,''/help/toolbox/simulink/help.jar!/slref/' lower(get_param(gcbh,'Blocktype')) '.html''], ''-helpbrowser''),end'])
      mask Display:
      | [x,y] = tlDrawBrandOnBlockIcon(gcbh);
      | plot(x,y);
  GreaterThan2 : RelationalOperator  RequirementInfo={} %GIDa_2ba9b958_4795_4006_aee4_e0e4590fb4e6  Operator=>  OutDataTypeStr=boolean  RndMeth=Nearest  mask(TL_RelationalOperator){data={'date',735992.65940515045}}
      settings: CopyFcn=if exist('copy_tlblock','file')==2,copy_tlblock(gcbh);end  DeleteFcn=if exist('delete_tlblock','file')==2,delete_tlblock(gcbh);end  NameChangeFcn=if exist('rename_tlblock','file')==2,rename_tlblock(gcbh);end  OpenFcn=if exist('tl_open_blockdlg','file')==2,tl_open_blockdlg(gcbh);else,open_system(gcbh,'parameter');end
      mask Help: eval(['if exist(''tl_online_help'',''file'') == 2, tl_online_help(''Topic'',''TL_RelationalOperator''),else, web([''jar:file:///'',matlabroot,''/help/toolbox/simulink/help.jar!/slref/' lower(get_param(gcbh,'Blocktype')) '.html''], ''-helpbrowser''),end'])
      mask Display:
      | [x,y] = tlDrawBrandOnBlockIcon(gcbh);
      | plot(x,y);
  Obstacle_off_value : Constant  RequirementInfo={} %GIDa_213879f6_1fdc_4138_9344_c6223ff2669e  Value=0  mask(TL_Constant){data={'date',735992.66084980324}}
      settings: CopyFcn=if exist('copy_tlblock','file')==2,copy_tlblock(gcbh);end  DeleteFcn=if exist('delete_tlblock','file')==2,delete_tlblock(gcbh);end  NameChangeFcn=if exist('rename_tlblock','file')==2,rename_tlblock(gcbh);end  OpenFcn=if exist('tl_open_blockdlg','file')==2,tl_open_blockdlg(gcbh);else,open_system(gcbh,'parameter');end
      mask Help: eval(['if exist(''tl_online_help'',''file'') == 2, tl_online_help(''Topic'',''TL_Constant''),else, web([''jar:file:///'',matlabroot,''/help/toolbox/simulink/help.jar!/slref/' lower(get_param(gcbh,'Blocktype')) '.html''], ''-helpbrowser''),end'])
      mask Display:
      | [x,y] = tlDrawBrandOnBlockIcon(gcbh);
      | plot(x,y);
  detection_obstacle : Logic  RequirementInfo={} %GIDa_16f10cb1_695d_4a90_9434_5f115b470f6c  AllPortsSameDT=off  OutDataTypeStr=boolean  mask(TL_LogicalOperator){data={'output',{'variable','Internal_Variables/detection_obstacle'},'date',738946.61777594907}}
      settings: CopyFcn=if exist('copy_tlblock','file')==2,copy_tlblock(gcbh);end  DeleteFcn=if exist('delete_tlblock','file')==2,delete_tlblock(gcbh);end  NameChangeFcn=if exist('rename_tlblock','file')==2,rename_tlblock(gcbh);end  OpenFcn=if exist('tl_open_blockdlg','file')==2,tl_open_blockdlg(gcbh);else,open_system(gcbh,'parameter');end
      mask Help: eval(['if exist(''tl_online_help'',''file'') == 2, tl_online_help(''Topic'',''TL_LogicalOperator''),else, web([''jar:file:///'',matlabroot,''/help/toolbox/simulink/help.jar!/slref/' lower(get_param(gcbh,'Blocktype')) '.html''], ''-helpbrowser''),end'])
      mask Display:
      | [x,y] = tlDrawBrandOnBlockIcon(gcbh);
      | plot(x,y);
  obstacle : Outport  RequirementInfo={} %GIDa_b08166f9_ff5c_44c2_9418_06c0e0e3d6bb  VectorParamsAs1DForOutWhenUnconnected=off
  wires:
  Obstacle_off_value/1 -> GreaterThan2/2
  obstacle_position/1 -> GreaterThan/2, GreaterThan2/1
  GreaterThan2/1 -> AND/2
  move_up/1 -> detection_obstacle/2
  AND/1 -> detection_obstacle/1  "obstacle_on_off"
  GreaterThan/1 -> AND/1
  window_position/1 -> GreaterThan/1
  detection_obstacle/1 -> obstacle/1  "obstacle_detection"

== system powerwindow_tl_v01/power_window_controller/Subsystem/power_window_controller/validate_driver/check_down ==
  action1 : Inport  RequirementInfo={} %GIDa_8734508f_23e0_4a4f_aca5_a826659845d5
  endstop1 : Inport  RequirementInfo={} %GIDa_905baa11_b4e5_4ab6_9444_79a1eb01194a  Port=2
  Terminator : Terminator
  checked_action1 : Outport  RequirementInfo={} %GIDa_c0b6f0c5_e7fa_4fba_9722_099ba5cb3bd6  VectorParamsAs1DForOutWhenUnconnected=off
  wires:
  action1/1 -> checked_action1/1
  endstop1/1 -> Terminator/1

== system powerwindow_tl_v01/power_window_controller/Subsystem/power_window_controller/validate_driver/check_up ==
  action : Inport  RequirementInfo={} %GIDa_1daa90c1_1a6f_4441_a241_f739eb12c7fb
  endstop : Inport  RequirementInfo={} %GIDa_74c191ec_ce33_4fc0_a067_b025c3a7629f  Port=2
  allow_action : Logic  RequirementInfo={} %GIDa_985b9295_c5bf_4850_9012_d4d583c40e79  AllPortsSameDT=off  OutDataTypeStr=boolean  mask(TL_LogicalOperator){data={'date',730486}}
      settings: CopyFcn=if exist('copy_tlblock','file')==2,copy_tlblock(gcbh);end  DeleteFcn=if exist('delete_tlblock','file')==2,delete_tlblock(gcbh);end  NameChangeFcn=if exist('rename_tlblock','file')==2,rename_tlblock(gcbh);end  OpenFcn=if exist('tl_open_blockdlg','file')==2,tl_open_blockdlg(gcbh);else,open_system(gcbh,'parameter');end
      mask Help: eval(['if exist(''tl_online_help'',''file'') == 2, tl_online_help(''Topic'',''TL_LogicalOperator''),else, web([''jar:file:///'',matlabroot,''/help/toolbox/simulink/help.jar!/slref/' lower(get_param(gcbh,'Blocktype')) '.html''], ''-helpbrowser''),end'])
      mask Display:
      | [x,y] = tlDrawBrandOnBlockIcon(gcbh);
      | plot(x,y);
  not : Logic  RequirementInfo={} %GIDa_84081eee_8376_475c_8d1e_e71ca41de5af  Operator=NOT  Inputs=1  AllPortsSameDT=off  OutDataTypeStr=boolean  mask(TL_LogicalOperator){data={'date',735992.62481011578}}
      settings: CopyFcn=if exist('copy_tlblock','file')==2,copy_tlblock(gcbh);end  DeleteFcn=if exist('delete_tlblock','file')==2,delete_tlblock(gcbh);end  NameChangeFcn=if exist('rename_tlblock','file')==2,rename_tlblock(gcbh);end  OpenFcn=if exist('tl_open_blockdlg','file')==2,tl_open_blockdlg(gcbh);else,open_system(gcbh,'parameter');end
      mask Help: eval(['if exist(''tl_online_help'',''file'') == 2, tl_online_help(''Topic'',''TL_LogicalOperator''),else, web([''jar:file:///'',matlabroot,''/help/toolbox/simulink/help.jar!/slref/' lower(get_param(gcbh,'Blocktype')) '.html''], ''-helpbrowser''),end'])
      mask Display:
      | [x,y] = tlDrawBrandOnBlockIcon(gcbh);
      | plot(x,y);
  checked_action : Outport  RequirementInfo={} %GIDa_5d869f0d_c393_4d33_8434_f495681cc19e  VectorParamsAs1DForOutWhenUnconnected=off
  wires:
  not/1 -> allow_action/2
  endstop/1 -> not/1
  action/1 -> allow_action/1
  allow_action/1 -> checked_action/1  "checked_action"

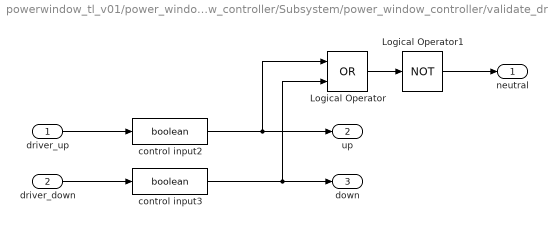
== system powerwindow_tl_v01/power_window_controller/Subsystem/power_window_controller/validate_driver/driver_switch ==
  driver_up : Inport  RequirementInfo={} %GIDa_88509d42_ace7_45cf_b2c2_89e39ae0ed2c
  driver_down : Inport  RequirementInfo={} %GIDa_beb14dc3_344f_4742_a2d0_fd6ea4a2bf32  Port=2
  Logical Operator : Logic  RequirementInfo={} %GIDa_da5550dd_f94c_4b73_b961_4a47a5203149  Operator=OR  AllPortsSameDT=off  OutDataTypeStr=boolean  mask(TL_LogicalOperator){data={'date',735992.62219250004}}
      settings: CopyFcn=if exist('copy_tlblock','file')==2,copy_tlblock(gcbh);end  DeleteFcn=if exist('delete_tlblock','file')==2,delete_tlblock(gcbh);end  NameChangeFcn=if exist('rename_tlblock','file')==2,rename_tlblock(gcbh);end  OpenFcn=if exist('tl_open_blockdlg','file')==2,tl_open_blockdlg(gcbh);else,open_system(gcbh,'parameter');end
      mask Help: eval(['if exist(''tl_online_help'',''file'') == 2, tl_online_help(''Topic'',''TL_LogicalOperator''),else, web([''jar:file:///'',matlabroot,''/help/toolbox/simulink/help.jar!/slref/' lower(get_param(gcbh,'Blocktype')) '.html''], ''-helpbrowser''),end'])
      mask Display:
      | [x,y] = tlDrawBrandOnBlockIcon(gcbh);
      | plot(x,y);
  Logical Operator1 : Logic  RequirementInfo={} %GIDa_999e8679_8f6d_4720_ab4a_29693e123b6b  Operator=NOT  Inputs=1  AllPortsSameDT=off  OutDataTypeStr=boolean  mask(TL_LogicalOperator){data={'date',735992.62266063655}}
      settings: CopyFcn=if exist('copy_tlblock','file')==2,copy_tlblock(gcbh);end  DeleteFcn=if exist('delete_tlblock','file')==2,delete_tlblock(gcbh);end  NameChangeFcn=if exist('rename_tlblock','file')==2,rename_tlblock(gcbh);end  OpenFcn=if exist('tl_open_blockdlg','file')==2,tl_open_blockdlg(gcbh);else,open_system(gcbh,'parameter');end
      mask Help: eval(['if exist(''tl_online_help'',''file'') == 2, tl_online_help(''Topic'',''TL_LogicalOperator''),else, web([''jar:file:///'',matlabroot,''/help/toolbox/simulink/help.jar!/slref/' lower(get_param(gcbh,'Blocktype')) '.html''], ''-helpbrowser''),end'])
      mask Display:
      | [x,y] = tlDrawBrandOnBlockIcon(gcbh);
      | plot(x,y);
  control input2 : DataTypeConversion  RequirementInfo={} %GIDa_1fd256de_8139_439f_b8bd_b0cd16c1aab9  OutDataTypeStr=boolean  SaturateOnIntegerOverflow=on  RndMeth=Zero  mask(TL_Rescaler){data={'date',730486}}
      settings: CopyFcn=if exist('copy_tlblock','file')==2,copy_tlblock(gcbh);end  DeleteFcn=if exist('delete_tlblock','file')==2,delete_tlblock(gcbh);end  NameChangeFcn=if exist('rename_tlblock','file')==2,rename_tlblock(gcbh);end  OpenFcn=if exist('tl_open_blockdlg','file')==2,tl_open_blockdlg(gcbh);else,open_system(gcbh,'parameter');end
      mask Help: eval(['if exist(''tl_online_help'',''file'') == 2, tl_online_help(''Topic'',''TL_Rescaler''),else, web([''jar:file:///'',matlabroot,''/help/toolbox/simulink/help.jar!/slref/' lower(get_param(gcbh,'Blocktype')) '.html''], ''-helpbrowser''),end'])
      mask Display:
      | [x,y] = tlDrawBrandOnBlockIcon(gcbh);
      | plot(x,y);
  control input3 : DataTypeConversion  RequirementInfo={} %GIDa_36784b95_c4a4_49da_bf15_3958bcd12f2f  OutDataTypeStr=boolean  SaturateOnIntegerOverflow=on  RndMeth=Zero  mask(TL_Rescaler){data={'date',730486}}
      settings: CopyFcn=if exist('copy_tlblock','file')==2,copy_tlblock(gcbh);end  DeleteFcn=if exist('delete_tlblock','file')==2,delete_tlblock(gcbh);end  NameChangeFcn=if exist('rename_tlblock','file')==2,rename_tlblock(gcbh);end  OpenFcn=if exist('tl_open_blockdlg','file')==2,tl_open_blockdlg(gcbh);else,open_system(gcbh,'parameter');end
      mask Help: eval(['if exist(''tl_online_help'',''file'') == 2, tl_online_help(''Topic'',''TL_Rescaler''),else, web([''jar:file:///'',matlabroot,''/help/toolbox/simulink/help.jar!/slref/' lower(get_param(gcbh,'Blocktype')) '.html''], ''-helpbrowser''),end'])
      mask Display:
      | [x,y] = tlDrawBrandOnBlockIcon(gcbh);
      | plot(x,y);
  neutral : Outport  RequirementInfo={} %GIDa_52397442_78d7_49fa_a893_524ae7078fcb  VectorParamsAs1DForOutWhenUnconnected=off
  up : Outport  RequirementInfo={} %GIDa_11ca0414_1b98_43c5_8236_d6cb17915be3  Port=2  VectorParamsAs1DForOutWhenUnconnected=off
  down : Outport  RequirementInfo={} %GIDa_c006668c_2a8f_411c_a55d_2fcf10c84114  Port=3  VectorParamsAs1DForOutWhenUnconnected=off
  wires:
  Logical Operator1/1 -> neutral/1
  Logical Operator/1 -> Logical Operator1/1
  control input3/1 -> Logical Operator/2, down/1
  control input2/1 -> Logical Operator/1, up/1
  driver_down/1 -> control input3/1
  driver_up/1 -> control input2/1
